simulink model "expert_3t"  (R2023a)
settings: Solver=VariableStepAuto  StartTime=0.0  StopTime=1000  RelTol=1e-3
values from neighbouring files (symbols this model uses):
  A = 0.0154    [parametros.m]    (also in variables.mat)
  az1 = 1    [parametros.m]    (also in variables.mat)
  az2 = 1    [parametros.m]    (also in variables.mat)
  az3 = 1    [parametros.m]    (also in variables.mat)
  g = 9.8    [parametros.m]    (also in variables.mat)
  H_star1 = 0.4    [parametros.m]    (also in variables.mat)
  H_star2 = 0.15    [parametros.m]    (also in variables.mat)
  Sn = 5e-5    (= 5e-05)    [parametros.m]    (also in variables.mat)
  st = 0.001    [parametros.m]    (also in variables.mat)
settings Model: Creator=empg0  LastModifiedBy=empg0

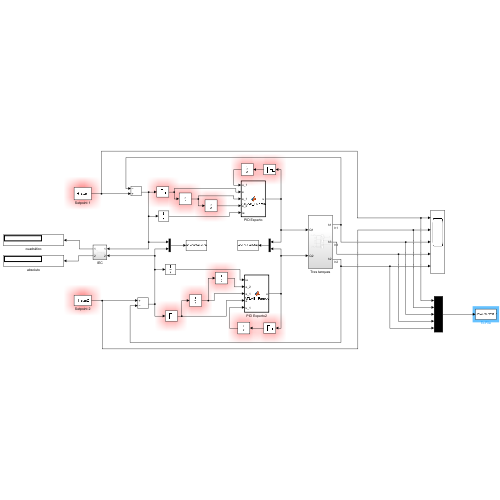
[thumbnail: Simulink's stored preview of the top-level diagram]
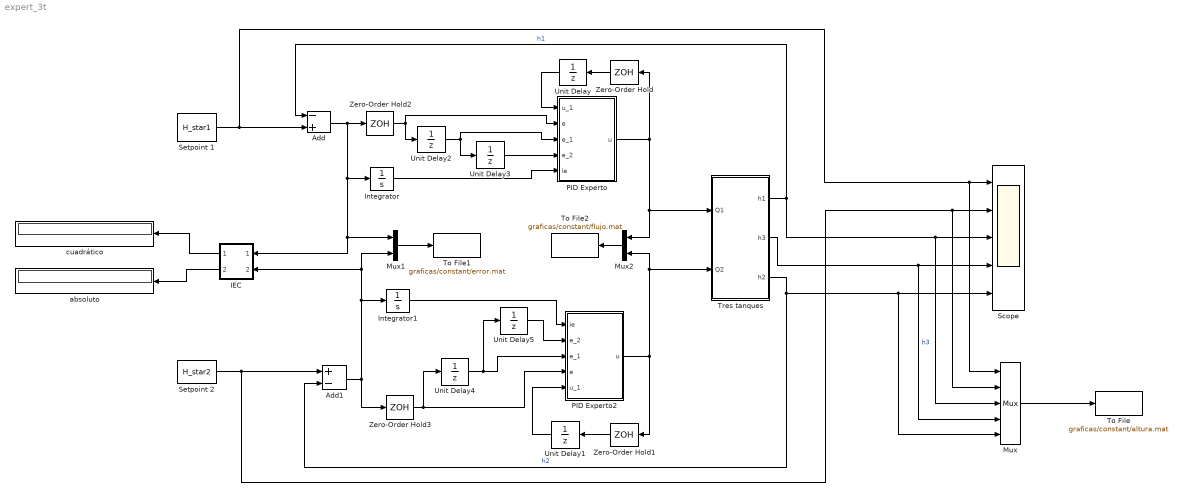
== system expert_3t ==
  Add : Sum  Inputs=-+
  Add1 : Sum  Inputs=+-
  IEC : Subsystem
  Integrator : Integrator
  Integrator1 : Integrator
  Mux : Mux  Inputs=5
  Mux1 : Mux  Inputs=2
  Mux2 : Mux  Inputs=2
  PID Experto : MATLAB Function  TreatAsAtomicUnit=on
  PID Experto2 : MATLAB Function  TreatAsAtomicUnit=on
  Scope : Scope  NumInputPorts=5
  Setpoint 1 : Constant  Value=H_star1
  Setpoint 2 : Constant  Value=H_star2
  To File : ToFile  Filename=graficas/constant/altura.mat  MatrixName=altura  SampleTime=0.5
  To File1 : ToFile  Filename=graficas/constant/error.mat  MatrixName=error  SampleTime=0.5
  To File2 : ToFile  Filename=graficas/constant/flujo.mat  MatrixName=flujo  SampleTime=0.5
  Tres tanques : Subsystem
  Unit Delay{,1..5} (6 alike) : UnitDelay  SampleTime=st  HasFrameUpgradeWarning=on
  Zero-Order Hold{,1..3} (4 alike) : ZeroOrderHold  SampleTime=st
  absoluto : Display
  cuadrático : Display
  wires:
  PID Experto/1(u) -> Tres tanques/1(Q1), Mux2/1, Zero-Order Hold/1
  Zero-Order Hold/1 -> Unit Delay/1
  Unit Delay/1 -> PID Experto/1(u_1)
  PID Experto2/1(u) -> Mux2/2, Tres tanques/2(Q2), Zero-Order Hold1/1
  Zero-Order Hold1/1 -> Unit Delay1/1
  Unit Delay1/1 -> PID Experto2/5(u_1)
  Setpoint 1/1 -> Mux/1, Scope/1, Add/2
  Tres tanques/1(h1) -> Add/1, Mux/3, Scope/3  "h1"
  Add/1 -> Mux1/1, IEC/1(In1), Integrator/1, Zero-Order Hold2/1
  Zero-Order Hold2/1 -> PID Experto/2(e), Unit Delay2/1
  Unit Delay2/1 -> PID Experto/3(e_1), Unit Delay3/1
  Unit Delay3/1 -> PID Experto/4(e_2)
  Integrator/1 -> PID Experto/5(ie)
  Setpoint 2/1 -> Mux/2, Scope/2, Add1/1
  Tres tanques/3(h2) -> Add1/2, Mux/5, Scope/5  "h2"
  Add1/1 -> Mux1/2, IEC/2(In2), Integrator1/1, Zero-Order Hold3/1
  Integrator1/1 -> PID Experto2/1(ie)
  Zero-Order Hold3/1 -> Unit Delay4/1, PID Experto2/4(e)
  Unit Delay5/1 -> PID Experto2/2(e_2)
  Unit Delay4/1 -> Unit Delay5/1, PID Experto2/3(e_1)
  Tres tanques/2(h3) -> Mux/4, Scope/4  "h3"
  IEC/1(Out1) -> cuadrático/1
  Mux/1 -> To File/1
  Mux1/1 -> To File1/1
  Mux2/1 -> To File2/1
  IEC/2(Out2) -> absoluto/1

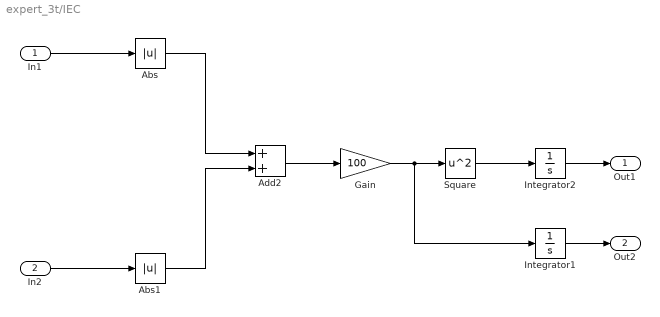
== system expert_3t/IEC ==
  In1 : Inport
  In2 : Inport  Port=2
  Abs : Abs  SaturateOnIntegerOverflow=off
  Abs1 : Abs  SaturateOnIntegerOverflow=off
  Add2 : Sum
  Gain : Gain  Gain=100
  Integrator1 : Integrator
  Integrator2 : Integrator
  Square : Math  Operator=square
  Out1 : Outport
  Out2 : Outport  Port=2
  wires:
  Abs1/1 -> Add2/2
  Abs/1 -> Add2/1
  In2/1 -> Abs1/1
  Square/1 -> Integrator2/1
  Integrator2/1 -> Out1/1
  In1/1 -> Abs/1
  Add2/1 -> Gain/1
  Gain/1 -> Integrator1/1, Square/1
  Integrator1/1 -> Out2/1

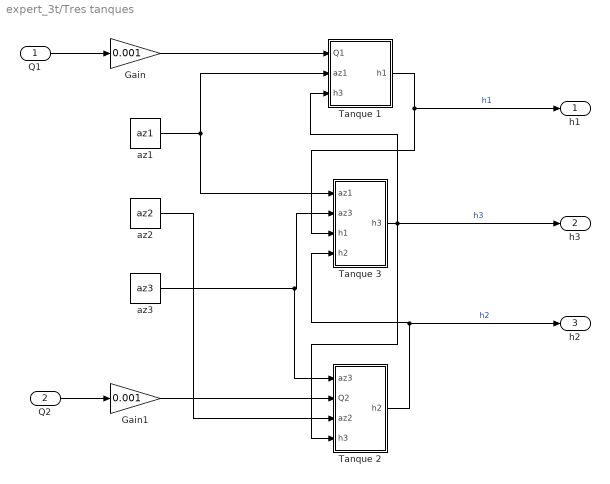
== system expert_3t/Tres tanques ==
  Q1 : Inport
  Q2 : Inport  Port=2
  Gain : Gain  Gain=0.001
  Gain1 : Gain  Gain=0.001
  Tanque 1 : Subsystem
  Tanque 2 : Subsystem
  Tanque 3 : Subsystem
  az1 : Constant  Value=az1
  az2 : Constant  Value=az2
  az3 : Constant  Value=az3
  h1 : Outport
  h3 : Outport  Port=2
  h2 : Outport  Port=3
  wires:
  Tanque 2/1(h2) -> Tanque 3/4(h2), h2/1  "h2"
  Tanque 1/1(h1) -> Tanque 3/3(h1), h1/1  "h1"
  Gain1/1 -> Tanque 2/2(Q2)
  Tanque 3/1(h3) -> Tanque 2/4(h3), h3/1, Tanque 1/3(h3)  "h3"
  az3/1 -> Tanque 2/1(az3), Tanque 3/2(az3)
  az1/1 -> Tanque 3/1(az1), Tanque 1/2(az1)
  az2/1 -> Tanque 2/3(az2)
  Gain/1 -> Tanque 1/1(Q1)
  Q1/1 -> Gain/1
  Q2/1 -> Gain1/1

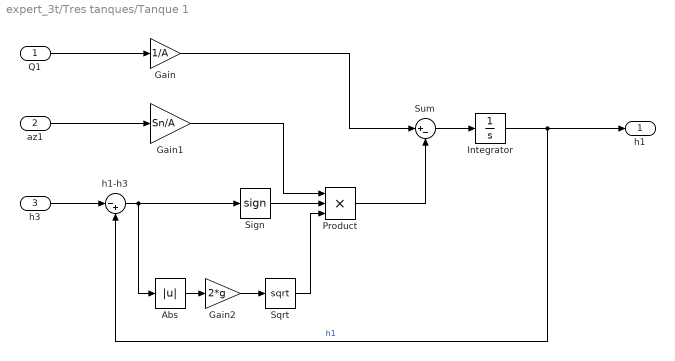
== system expert_3t/Tres tanques/Tanque 1 ==
  Q1 : Inport
  az1 : Inport  Port=2
  h3 : Inport  Port=3
  Abs : Abs  SaturateOnIntegerOverflow=off
  Gain : Gain  Gain=1/A
  Gain1 : Gain  Gain=Sn/A
  Gain2 : Gain  Gain=2*g
  Integrator : Integrator  LimitOutput=on  UpperSaturationLimit=0.62  LowerSaturationLimit=0
  Product : Product  Inputs=3
  Sign : Signum
  Sqrt : Sqrt
  Sum : Sum  Inputs=|+-
  h1-h3 : Sum  Inputs=|-+
  h1 : Outport
  wires:
  h3/1 -> h1-h3/1
  Sum/1 -> Integrator/1
  Gain2/1 -> Sqrt/1
  Gain1/1 -> Product/1
  Sqrt/1 -> Product/3
  Sign/1 -> Product/2
  h1-h3/1 -> Abs/1, Sign/1
  Q1/1 -> Gain/1
  az1/1 -> Gain1/1
  Integrator/1 -> h1/1, h1-h3/2  "h1"
  Product/1 -> Sum/2
  Gain/1 -> Sum/1
  Abs/1 -> Gain2/1

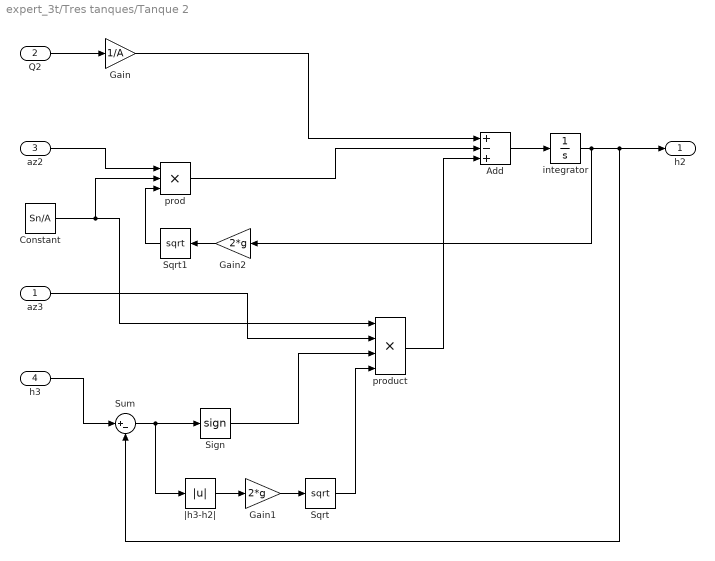
== system expert_3t/Tres tanques/Tanque 2 ==
  az3 : Inport
  Q2 : Inport  Port=2
  az2 : Inport  Port=3
  h3 : Inport  Port=4
  Add : Sum  Inputs=+-+
  Constant : Constant  Value=Sn/A
  Gain : Gain  Gain=1/A
  Gain1 : Gain  Gain=2*g
  Gain2 : Gain  Gain=2*g
  Sign : Signum
  Sqrt : Sqrt
  Sqrt1 : Sqrt
  Sum : Sum  Inputs=|+-
  integrator : Integrator  LimitOutput=on  UpperSaturationLimit=0.62  LowerSaturationLimit=0
  prod : Product  Inputs=3
  product : Product  Inputs=4
  |h3-h2| : Abs  SaturateOnIntegerOverflow=off
  h2 : Outport
  wires:
  |h3-h2|/1 -> Gain1/1
  prod/1 -> Add/2
  product/1 -> Add/3
  Add/1 -> integrator/1
  Gain/1 -> Add/1
  Constant/1 -> product/1, prod/2
  Gain1/1 -> Sqrt/1
  Sum/1 -> |h3-h2|/1, Sign/1
  az2/1 -> prod/1
  az3/1 -> product/2
  Sqrt1/1 -> prod/3
  Sqrt/1 -> product/4
  Sign/1 -> product/3
  h3/1 -> Sum/1
  integrator/1 -> Gain2/1, h2/1, Sum/2
  Gain2/1 -> Sqrt1/1
  Q2/1 -> Gain/1

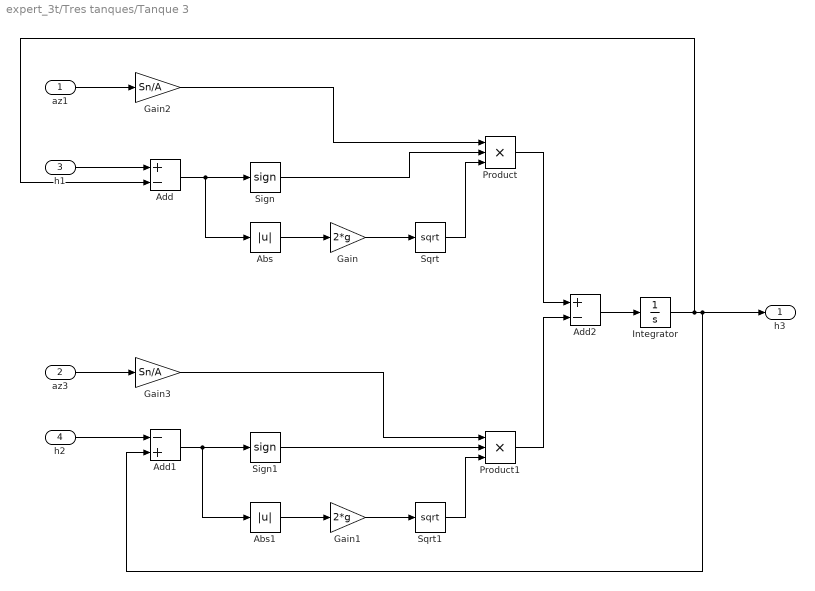
== system expert_3t/Tres tanques/Tanque 3 ==
  az1 : Inport
  az3 : Inport  Port=2
  h1 : Inport  Port=3
  h2 : Inport  Port=4
  Abs : Abs  SaturateOnIntegerOverflow=off
  Abs1 : Abs  SaturateOnIntegerOverflow=off
  Add : Sum  Inputs=+-
  Add1 : Sum  Inputs=-+
  Add2 : Sum  Inputs=+-
  Gain : Gain  Gain=2*g
  Gain1 : Gain  Gain=2*g
  Gain2 : Gain  Gain=Sn/A
  Gain3 : Gain  Gain=Sn/A
  Integrator : Integrator  LimitOutput=on  UpperSaturationLimit=0.62  LowerSaturationLimit=0
  Product : Product  Inputs=3
  Product1 : Product  Inputs=3
  Sign : Signum
  Sign1 : Signum
  Sqrt : Sqrt
  Sqrt1 : Sqrt
  h3 : Outport
  wires:
  Add2/1 -> Integrator/1
  Gain3/1 -> Product1/1
  az1/1 -> Gain2/1
  Gain1/1 -> Sqrt1/1
  Add1/1 -> Abs1/1, Sign1/1
  h1/1 -> Add/1
  az3/1 -> Gain3/1
  Integrator/1 -> h3/1, Add1/2, Add/2
  Abs1/1 -> Gain1/1
  Add/1 -> Abs/1, Sign/1
  Abs/1 -> Gain/1
  Sqrt1/1 -> Product1/3
  Sign/1 -> Product/2
  Product1/1 -> Add2/2
  Gain2/1 -> Product/1
  Sqrt/1 -> Product/3
  Sign1/1 -> Product1/2
  Gain/1 -> Sqrt/1
  h2/1 -> Add1/1
  Product/1 -> Add2/1

== matlab function expert_3t/PID Experto ==
  data: u_1 input; e input; u output; e_1 input; e_2 input; ie input
function u = MATLAB_Function(u_1, e, e_1, e_2, ie)
    
    %st = load("sampling_time.mat");
    % Constantes
    H_max = 0.62;
    M1 = H_max/2;
    M2 = H_max/4;
    epsilon = 0.001; % cambié de 0.01 a 0.005
    st = 0.001; % 0.1 -> 0.001

    Qmax = 0.1; % flujo máximo
    Qmin = 0; % flujo mínimo
    
    k1 = 4.9321;
    k2 = 0.033265;
    kp = 1.06160;
    ki = 0.05; %0.03014;
    kd = -2.20023;

    de = e - e_1;
    de_1 = e_1 - e_2;
    if abs(e) > M1 % regla 1
        r = 1;
        if e > 0
            u = Qmax;
        else
            u = Qmin;
        end
    elseif abs(e) <= epsilon % regla 5
        r = 5;
        u = u_1 + kp*(e - e_1) + ki*ie;
    elseif e*de < 0 && de*de_1 < 0 % regla 4
        r = 4;
        if abs(e) >= M2
            u = u_1 + k1*kp*e;
        else
            u = u_1 + k2*kp*e;
        end
    elseif (e*de < 0 && de*de_1 > 0) || e == 0 % regla 3
        r = 3;
        u = u_1;
    elseif e*de > 0 || de == 0 % regla 2
        % funcionaba mejor cuando la regla 2 era pid normal
        r = 2;
        if abs(e) >= M2
            %control fuerte
            u = u_1 + k1*kp*(e - e_1) + k1*ki*e + k1*kd*(e - 2*e_1 + e_2);
        else
            %control débil
            u = u_1 + kp*(e - e_1) + ki*e + kd*(e - 2*e_1 + e_2);
        end
    else
        r = 0;
        u = kp*e + (kd*de)/st + ki*ie;
    end
    if u > 0.1
        u = 0.1;
    end
    if u < 0
        u = 0;
    end

== matlab function expert_3t/PID Experto2 ==
  data: ie input; e_2 input; e_1 input; e input; u_1 input; u output
function u = MATLAB_Function(ie, e_2, e_1, e, u_1)
    
    %st = load("sampling_time.mat");
    % Constantes
    H_max = 0.62;
    M1 = H_max/3;
    M2 = H_max/6;
    epsilon = 0.001;
    st = 0.001;

    Qmax = 0.1; % flujo máximo
    Qmin = 0; % flujo mínimo
    
    k1 = 4.9321;
    k2 = 0.033265;
    kp = 1.06160;
    ki = 0.05; %0.03014;
    kd = -2.20023;

    de = e - e_1;
    de_1 = e_1 - e_2;
    if abs(e) > M1 % regla 1
        r = 1;
        if e > 0
            u = Qmax;
        else
            u = Qmin;
        end
    elseif abs(e) <= epsilon % regla 5
        r = 5;
        u = u_1 + kp*(e - e_1) + ki*ie;
    elseif e*de < 0 && de*de_1 < 0 % regla 4
        r = 4;
        if abs(e) >= M2
            u = u_1 + k1*kp*e;
        else
            u = u_1 + k2*kp*e;
        end
    elseif (e*de < 0 && de*de_1 > 0) || e == 0 % regla 3
        r = 3;
        u = u_1;
    elseif e*de > 0 || de == 0 % regla 2
        % funcionaba mejor cuando la regla 2 era pid normal
        r = 2;
        if abs(e) >= M2
            %control fuerte
            u = u_1 + k1*kp*(e - e_1) + k1*ki*e + k1*kd*(e - 2*e_1 + e_2);
        else
            %control débil
            u = u_1 + kp*(e - e_1) + ki*e + kd*(e - 2*e_1 + e_2);
        end
    else
        r = 0;
        u = kp*e + (kd*de)/st + ki*ie;
    end
    if u > 0.1
        u = 0.1;
    end
    if u < 0
        u = 0;
    end
